simulink model "viphough"  (R2015b)
settings: Solver=FixedStepDiscrete  StartTime=0.0  StopTime=inf  RelTol=1e-3
undefined symbols (not defined in the file or in its folder): gray, hot, strel
libraries: visionsinks x4, visiongeotforms x3, visionstatistics x3, visionmorphops x2, vipmisc x1, visionsources x1, visiontransforms x1
settings Model: FPTRunName=Active  Creator=The MathWorks, Inc.  LastModifiedBy=The MathWorks, Inc.
settings DataIOCC: SaveFormat=Array
settings OptimizationCC: ExpressionDepthLimit=2147483647  InitFltsAndDblsToZero=on
settings DebuggingCC: UnderspecifiedInitializationDetection=Classic  MergeDetectMultiDrivingBlocksExec=none  SignalResolutionControl=TryResolveAllWithWarning  SolverPrmCheckMsg=warning  MultiTaskDSMMsg=warning  MultiTaskCondExecSysMsg=none  FcnCallInpInsideContextMsg=UseLocalSettings  StateNameClashWarn=warning  StrictBusMsg=None
settings HardwareCC: ProdBitPerPointer=32  ProdLargestAtomicFloat=None  ProdIntDivRoundTo=Undefined  ProdEndianess=Unspecified  ProdWordSize=32  ProdHWDeviceType=32-bit Generic
settings SFSimCC: SimParseCustomCode=off
settings GRTTargetCC: TargetFcnLib=ansi_tfl_tmw_new.mat  GeneratePreprocessorConditionals=Disable all  CombineOutputUpdateFcns=off  GRTInterface=on
settings ConfigComp: CovModelRefEnable=Off

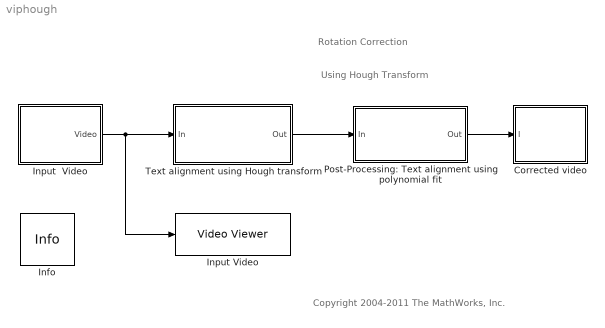
== system viphough ==
  note: Rotation Correction
  note: Using Hough Transform
  note: Copyright 2004-2011 The MathWorks, Inc.
  Corrected video : Subsystem
      mask Display:
      | disp('Video\nViewer');
      | port_label('input',1,'I');
  Info : vipmisc/Info  SystemSampleTime=-1
  Input  Video : Subsystem
  Input Video : visionsinks/Video Viewer  inputType=Obsolete7b  imagePorts=One multidimensional signal  useColorMap=off  colormapValue=gray(256)  specRange=off  minInputVal=0  maxInputVal=255  FigPos=[216 352 223 251]  AxisZoom=on  trueSizedOnce=on  OpenAtMdlStart=on  DefaultConfigurationName=vipscopes.VideoViewerScopeCfg
  Post-Processing: Text alignment using polynomial fit : Subsystem
  Text alignment using Hough transform : Subsystem
  wires:
  Post-Processing: Text alignment using polynomial fit/1(Out) -> Corrected video/1(I)
  Input  Video/1(Video) -> Text alignment using Hough transform/1(In), Input Video/1
  Text alignment using Hough transform/1(Out) -> Post-Processing: Text alignment using polynomial fit/1(In)

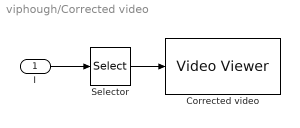
== system viphough/Corrected video ==
  I : Inport
  Corrected video : visionsinks/Video Viewer  inputType=Obsolete7b  imagePorts=One multidimensional signal  useColorMap=off  colormapValue=gray(256)  specRange=off  minInputVal=0  maxInputVal=255  FigPos=[701 355 221 254]  AxisZoom=on  trueSizedOnce=on  OpenAtMdlStart=on  DefaultConfigurationName=vipscopes.VideoViewerScopeCfg
  Selector : Selector  NumberOfDimensions=2  InputPortWidth=3  IndexOptions=Index vector (dialog),Index vector (dialog)  Indices=[112:(442-111)],[112:(442-111)]  OutputSizes=1,1
  wires:
  I/1 -> Selector/1
  Selector/1 -> Corrected video/1

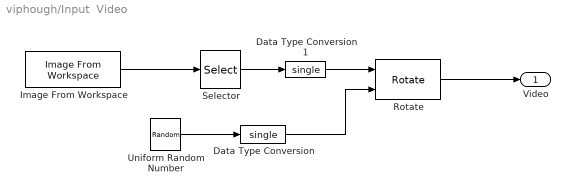
== system viphough/Input  Video ==
  Data Type Conversion1 : DataTypeConversion  OutDataTypeStr=single  SaturateOnIntegerOverflow=on  RndMeth=Zero
  Data Type Conversion : DataTypeConversion  OutDataTypeStr=single
  Image From Workspace : visionsources/Image From Workspace  Tag=vipblks_nd  ImageValue=imread('text.png')  Ts=inf  imagePorts=Separate color signals  ImageDataType=Inherit from 'Value'  Signed=on  WordLength=16  sdImageDataType=sfix(16)  FractionLengthMode=User-defined  FractionLength=15  OutPortLabels=I
  Rotate : visiongeotforms/Rotate  outSizeR=Expanded to fit rotated input image  src_angle=Input port  unit_angle=Degrees  angle=30  maxAngle=single(pi)  dispImage=Center  method=Table lookup  fillVal=0  interpMethod=Bilinear  prodOutputMode=Binary point scaling  prodOutputWordLength=32  prodOutputFracLength=16  roundingMode=Floor  overflowMode=off
  Selector : Selector  NumberOfDimensions=2  InputPortWidth=3  IndexOptions=Index vector (dialog),Index vector (dialog)  Indices=[5:60],[5:(256-40)]  OutputSizes=1,1
  Uniform Random Number : UniformRandomNumber  Minimum=-pi/6  Maximum=pi/6  SampleTime=1/30  VectorParams1D=off
  Video : Outport
  wires:
  Image From Workspace/1 -> Selector/1
  Data Type Conversion1/1 -> Rotate/1
  Selector/1 -> Data Type Conversion1/1
  Rotate/1 -> Video/1
  Uniform Random Number/1 -> Data Type Conversion/1
  Data Type Conversion/1 -> Rotate/2

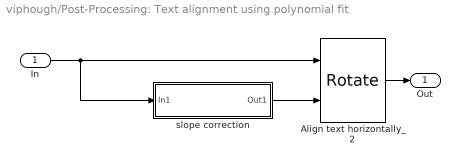
== system viphough/Post-Processing: Text alignment using polynomial fit ==
  In : Inport
  Align text horizontally_2 : visiongeotforms/Rotate  outSizeR=Expanded to fit rotated input image  src_angle=Input port  unit_angle=Radians  angle=30  maxAngle=single(pi)  dispImage=Center  method=Table lookup  fillVal=0  interpMethod=Bilinear  prodOutputMode=Binary point scaling  prodOutputWordLength=32  prodOutputFracLength=16  roundingMode=Floor  overflowMode=off
  slope correction : Subsystem
  Out : Outport
  wires:
  In/1 -> slope correction/1(In1), Align text horizontally_2/1
  slope correction/1(Out1) -> Align text horizontally_2/2
  Align text horizontally_2/1 -> Out/1

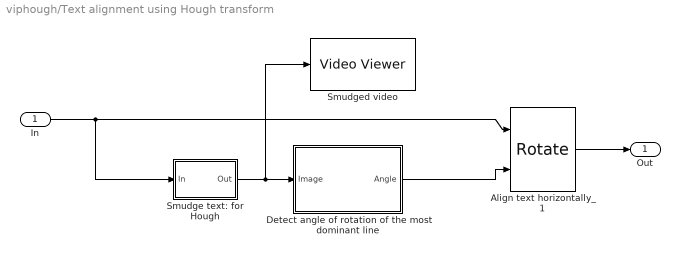
== system viphough/Text alignment using Hough transform ==
  In : Inport
  Align text horizontally_1 : visiongeotforms/Rotate  outSizeR=Expanded to fit rotated input image  src_angle=Input port  unit_angle=Radians  angle=30  maxAngle=single(pi)  dispImage=Center  method=Table lookup  fillVal=0  interpMethod=Bilinear  prodOutputMode=Binary point scaling  prodOutputWordLength=32  prodOutputFracLength=16  roundingMode=Floor  overflowMode=off
  Detect angle of rotation of the most dominant line : Subsystem
  Smudge text: for Hough : Subsystem
  Smudged video : visionsinks/Video Viewer  inputType=Obsolete7b  imagePorts=One multidimensional signal  useColorMap=off  colormapValue=gray(256)  specRange=off  minInputVal=0  maxInputVal=255  FigPos=[458 351 225 250]  AxisZoom=on  trueSizedOnce=on  OpenAtMdlStart=on  DefaultConfigurationName=vipscopes.VideoViewerScopeCfg
  Out : Outport
  wires:
  In/1 -> Smudge text: for Hough/1(In), Align text horizontally_1/1
  Detect angle of rotation of the most dominant line/1(Angle) -> Align text horizontally_1/2
  Smudge text: for Hough/1(Out) -> Detect angle of rotation of the most dominant line/1(Image), Smudged video/1
  Align text horizontally_1/1 -> Out/1

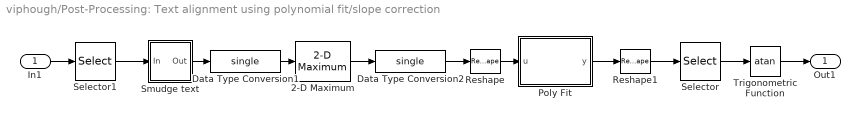
== system viphough/Post-Processing: Text alignment using polynomial fit/slope correction ==
  In1 : Inport
  2-D Maximum : visionstatistics/2-D Maximum  fcn=Index  reset=None  indexBase=One  operateOver=Each column  Dimension=1  colComp=on  operation=maximum  roiEnable=off  roiType=Rectangles  roiPortion=Entire ROI  roiOutput=Individual statistics for each ROI  roiFlag=off  accumDataTypeStr=Inherit: Same as product output  accumLastDataTypeStr=Inherit: Same as product output  roundingMode=Floor  overflowMode=off
  Data Type Conversion1 : DataTypeConversion  OutDataTypeStr=single  SaturateOnIntegerOverflow=on  RndMeth=Zero
  Data Type Conversion2 : DataTypeConversion  OutDataTypeStr=single  SaturateOnIntegerOverflow=on  RndMeth=Zero
  Poly Fit : MATLAB Function  TreatAsAtomicUnit=on
  Reshape : Reshape  OutputDimensionality=Column vector (2-D)
  Reshape1 : Reshape  OutputDimensionality=Column vector (2-D)
  Selector : Selector  InputPortWidth=2  IndexOptions=Index vector (dialog)  Indices=1  OutputSizes=1
  Selector1 : Selector  NumberOfDimensions=2  InputPortWidth=3  IndexOptions=Index vector (dialog),Index vector (dialog)  Indices=[100:(313-100)],[55:(313-75)]  OutputSizes=1,1
  Smudge text : Subsystem
  Trigonometric Function : Trigonometry  Operator=atan
  Out1 : Outport
  wires:
  Selector1/1 -> Smudge text/1(In)
  Selector/1 -> Trigonometric Function/1
  Trigonometric Function/1 -> Out1/1
  Reshape/1 -> Poly Fit/1(u)
  Smudge text/1(Out) -> Data Type Conversion1/1
  In1/1 -> Selector1/1
  Data Type Conversion1/1 -> 2-D Maximum/1
  Data Type Conversion2/1 -> Reshape/1
  2-D Maximum/1 -> Data Type Conversion2/1
  Poly Fit/1(y) -> Reshape1/1
  Reshape1/1 -> Selector/1

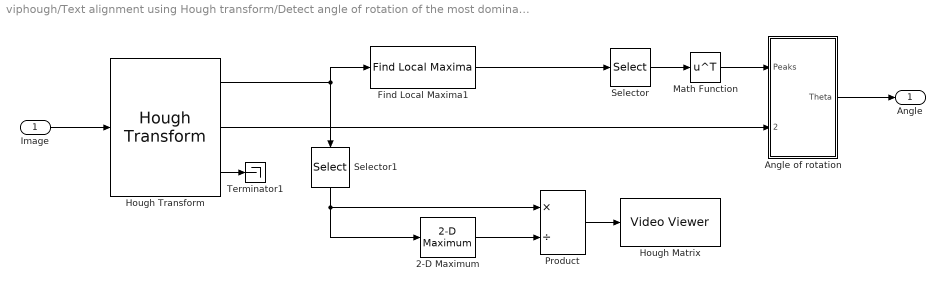
== system viphough/Text alignment using Hough transform/Detect angle of rotation of the most dominant line ==
  Image : Inport
  2-D Maximum : visionstatistics/2-D Maximum  fcn=Value  reset=None  indexBase=One  operateOver=Entire input  Dimension=1  colComp=on  operation=maximum  roiEnable=off  roiType=Rectangles  roiPortion=Entire ROI  roiOutput=Individual statistics for each ROI  roiFlag=off  accumDataTypeStr=Inherit: Same as product output  accumLastDataTypeStr=Inherit: Same as product output  roundingMode=Floor  overflowMode=off
  Angle of rotation : Subsystem
  Find Local Maxima1 : visionstatistics/Find Local Maxima  num_peaks=5  nhood_size=[21 11]  src_thresh=Obsolete9b  src_thresh_inuse=Specify via dialog  threshold=6  inputIsHough=on  dt_peak=single  isOutVarDim=on  dt_count=uint32
  Hough Matrix : visionsinks/Video Viewer  inputType=Obsolete7b  imagePorts=One multidimensional signal  useColorMap=on  colormapValue=hot(256);  specRange=off  minInputVal=0  maxInputVal=255  FigPos=[13 588 185 459]  AxisZoom=on  trueSizedOnce=on  OpenAtMdlStart=on  DefaultConfigurationName=vipscopes.VideoViewerScopeCfg
  Hough Transform : visiontransforms/Hough Transform  theta_res=(pi/180)  rho_res=1  out_theta_rho=on  outdtmode=single  firstCoeffMode=Binary point scaling  firstCoeffWordLength=16  firstCoeffFracLength=14  secondCoeffMode=Binary point scaling  secondCoeffWordLength=32  secondCoeffFracLength=16  outputMode=Binary point scaling  outputWordLength=16  outputFracLength=0  accumMode=Binary point scaling  accumWordLength=32  accumFracLength=20  prodOutputMode=Binary point scaling  prodOutputWordLength=32  prodOutputFracLength=20  memoryMode=Binary point scaling  memoryWordLength=32  memoryFracLength=16  roundingMode=Nearest  overflowMode=on
  Math Function : Math  Operator=transpose  SaturateOnIntegerOverflow=on
  Product : Product  Inputs=*/  SaturateOnIntegerOverflow=on  InputSameDT=on  OutDataTypeStr=Inherit: Same as first input
  Selector : Selector  NumberOfDimensions=2  InputPortWidth=3  IndexOptions=Select all,Index vector (dialog)  Indices=[1 3],[2 1]  OutputSizes=1,1
  Selector1 : Selector  NumberOfDimensions=2  InputPortWidth=3  IndexOptions=Index vector (dialog),Select all  Indices=[120:(621-70)],[112:(442-111)]  OutputSizes=1,1
  Terminator1 : Terminator
  Angle : Outport
  wires:
  Hough Transform/1 -> Find Local Maxima1/1, Selector1/1
  Hough Transform/2 -> Angle of rotation/2(Thetas)
  Hough Transform/3 -> Terminator1/1
  Image/1 -> Hough Transform/1
  Angle of rotation/1(Theta) -> Angle/1
  2-D Maximum/1 -> Product/2
  Product/1 -> Hough Matrix/1
  Selector1/1 -> Product/1, 2-D Maximum/1
  Find Local Maxima1/1 -> Selector/1
  Selector/1 -> Math Function/1
  Math Function/1 -> Angle of rotation/1(Peaks)

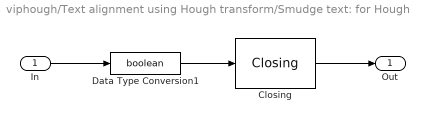
== system viphough/Text alignment using Hough transform/Smudge text: for Hough ==
  In : Inport
  Closing : visionmorphops/Closing  nhoodsrc=Specify via dialog  strel=strel('disk',4)
  Data Type Conversion1 : DataTypeConversion  OutDataTypeStr=boolean  SaturateOnIntegerOverflow=on  RndMeth=Zero
  Out : Outport
  wires:
  In/1 -> Data Type Conversion1/1
  Closing/1 -> Out/1
  Data Type Conversion1/1 -> Closing/1

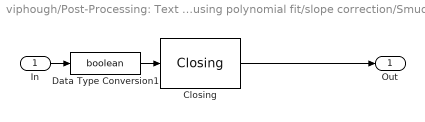
== system viphough/Post-Processing: Text alignment using polynomial fit/slope correction/Smudge text ==
  In : Inport
  Closing : visionmorphops/Closing  nhoodsrc=Specify via dialog  strel=strel('disk',4)
  Data Type Conversion1 : DataTypeConversion  OutDataTypeStr=boolean  SaturateOnIntegerOverflow=on  RndMeth=Zero
  Out : Outport
  wires:
  Closing/1 -> Out/1
  In/1 -> Data Type Conversion1/1
  Data Type Conversion1/1 -> Closing/1

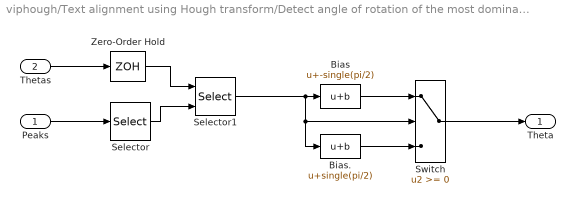
== system viphough/Text alignment using Hough transform/Detect angle of rotation of the most dominant line/Angle of rotation ==
  Peaks : Inport
  Thetas : Inport  Port=2
  Bias : Bias  Bias=-single(pi/2)
  Bias. : Bias  Bias=single(pi/2)
  Selector : Selector  NumberOfDimensions=2  InputPortWidth=3  IndexOptions=Index vector (dialog),Index vector (dialog)  Indices=2,1  OutputSizes=1
  Selector1 : Selector  NumberOfDimensions=2  InputPortWidth=3  IndexOptions=Select all,Index vector (port)  Indices=[1 3],1  OutputSizes=1,1
  Switch : Switch  InputSameDT=on
  Zero-Order Hold : ZeroOrderHold  SampleTime=-1
  Theta : Outport
  wires:
  Selector1/1 -> Bias/1, Bias./1, Switch/2
  Selector/1 -> Selector1/2
  Thetas/1 -> Zero-Order Hold/1
  Peaks/1 -> Selector/1
  Bias/1 -> Switch/1
  Bias./1 -> Switch/3
  Switch/1 -> Theta/1
  Zero-Order Hold/1 -> Selector1/1

== matlab function viphough/Post-Processing: Text alignment using polynomial fit/slope correction/Poly Fit ==
  data: u input; y output
function y = fcn(u)
%#codegen

x = (0:183)';

coeff = polyfit(x,u,1);
y=coeff';
